simulink model "reset_demo"  (R2015a)
settings: Solver=ode45  SolverMode=SingleTasking  StartTime=0.0  StopTime=100  RelTol=1e-3
libraries: simulink x2
settings Model: CovMetricSettings=dwe  CovHtmlReporting=off  covSaveCumulativeToWorkspaceVar=off  CovSaveSingleToWorkspaceVar=off  CovExternalEMLEnable=on  Creator=cbrooks  LastModifiedBy=hbourbou
settings DataIOCC: LimitDataPoints=off  SaveFormat=Dataset
settings DebuggingCC: SFUnexpectedBacktrackingDiag=error  SFNoUnconditionalDefaultTransitionDiag=error
settings HardwareCC: ProdBitPerPointer=64  ProdLargestAtomicFloat=Float  ProdIntDivRoundTo=Zero  ProdEndianess=LittleEndian  ProdHWDeviceType=Specified
settings ModelReferenceCC: PropagateSignalLabelsOutOfModel=on
settings GRTTargetCC: TargetLangStandard=C99 (ISO)  GeneratePreprocessorConditionals=Use local settings

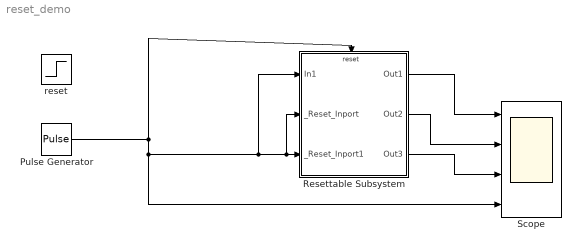
== system reset_demo ==
  Pulse Generator : DiscretePulseGenerator  Period=6  PulseWidth=3
  Resettable Subsystem : Subsystem  TreatAsAtomicUnit=on
  Scope : Scope  NumInputPorts=4
      settings: TimeRange=auto  MaxDataPoints=5000  SaveToWorkspace=off  SaveName=ScopeData  YMin=-0.375~-0.375~-0.375~-0.375  YMax=3.375~3.375~3.375~3.375  SampleTime=-1
  reset : Step  Time=5  SampleTime=.2
  wires:
  Pulse Generator/1 -> Resettable Subsystem/Reset, Scope/4, Resettable Subsystem/1(In1), Resettable Subsystem/2(_Reset_Inport), Resettable Subsystem/3(_Reset_Inport1)
  Resettable Subsystem/1(Out1) -> Scope/1
  Resettable Subsystem/3(Out3) -> Scope/3
  Resettable Subsystem/2(Out2) -> Scope/2

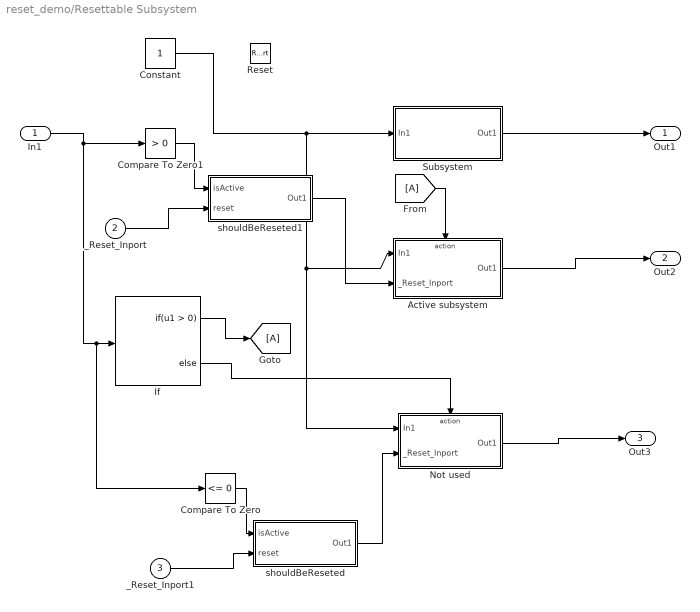
== system reset_demo/Resettable Subsystem ==
  In1 : Inport
  _Reset_Inport : Inport  Port=2
  _Reset_Inport1 : Inport  Port=3
  Reset : ResetPort  DisableCoverage=on  ResetTriggerType=level hold
  Active subsystem : Subsystem  TreatAsAtomicUnit=on
  Compare To Zero : simulink/Logic and Bit Operations/Compare To Zero  relop=<=  OutDataTypeStr=boolean
  Compare To Zero1 : simulink/Logic and Bit Operations/Compare To Zero  relop=>  OutDataTypeStr=boolean
  Constant : Constant  SampleTime=1
  If : If
  Not used : Subsystem  TreatAsAtomicUnit=on
  Subsystem : Subsystem
  shouldBeReseted : Subsystem
  shouldBeReseted1 : Subsystem
  Out1 : Outport
  Out2 : Outport  Port=2
  Out3 : Outport  Port=3
  wires:
  Constant/1 -> Subsystem/1(In1), Not used/1(In1), Active subsystem/1(In1)
  Active subsystem/1(Out1) -> Out2/1
  Subsystem/1(Out1) -> Out1/1
  If/1 -> [A]
  [A] -> Active subsystem/Action
  If/2 -> Not used/Action
  _Reset_Inport/1 -> shouldBeReseted1/2(reset)
  _Reset_Inport1/1 -> shouldBeReseted/2(reset)
  Not used/1(Out1) -> Out3/1
  Compare To Zero/1 -> shouldBeReseted/1(isActive)
  shouldBeReseted/1(Out1) -> Not used/2(_Reset_Inport)
  shouldBeReseted1/1(Out1) -> Active subsystem/2(_Reset_Inport)
  In1/1 -> Compare To Zero1/1, Compare To Zero/1, If/1
  Compare To Zero1/1 -> shouldBeReseted1/1(isActive)

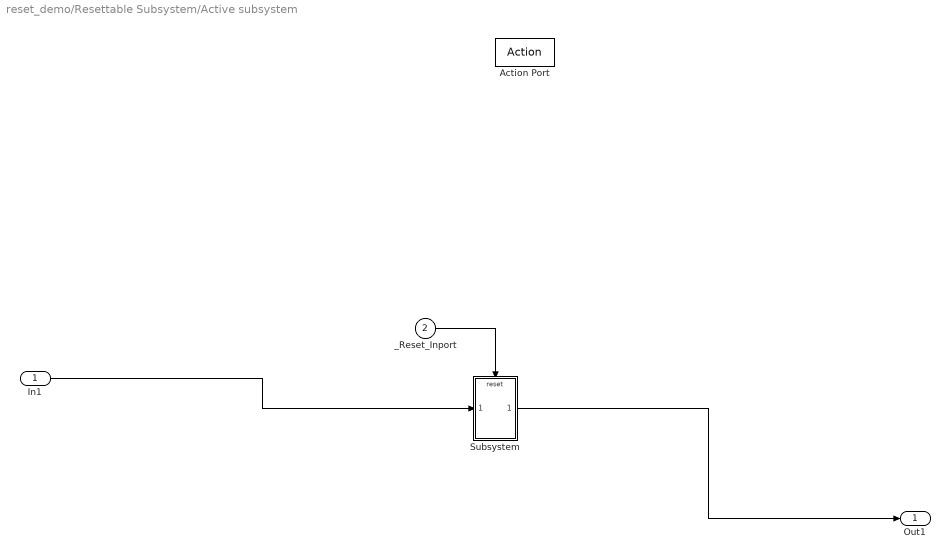
== system reset_demo/Resettable Subsystem/Active subsystem ==
  In1 : Inport
  _Reset_Inport : Inport  Port=2
  Action Port : ActionPort  ActionType=then
  Subsystem : Subsystem
  Out1 : Outport
  wires:
  In1/1 -> Subsystem/1(In1)
  Subsystem/1(Out1) -> Out1/1
  _Reset_Inport/1 -> Subsystem/Reset

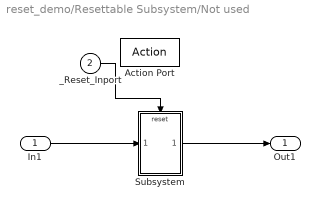
== system reset_demo/Resettable Subsystem/Not used ==
  In1 : Inport
  _Reset_Inport : Inport  Port=2
  Action Port : ActionPort  ActionType=else
  Subsystem : Subsystem
  Out1 : Outport
  wires:
  In1/1 -> Subsystem/1(In1)
  Subsystem/1(Out1) -> Out1/1
  _Reset_Inport/1 -> Subsystem/Reset

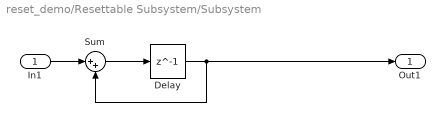
== system reset_demo/Resettable Subsystem/Subsystem ==
  In1 : Inport
  Delay : Delay  DelayLength=1
  Sum : Sum  Inputs=|++
  Out1 : Outport
  wires:
  Delay/1 -> Out1/1, Sum/2
  Sum/1 -> Delay/1
  In1/1 -> Sum/1

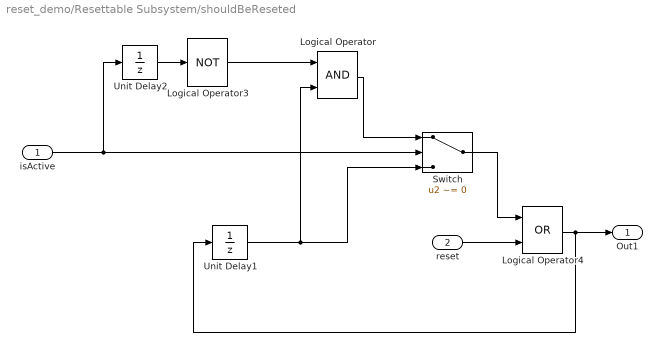
== system reset_demo/Resettable Subsystem/shouldBeReseted ==
  isActive : Inport
  reset : Inport  Port=2
  Logical Operator : Logic  AllPortsSameDT=off  OutDataTypeStr=boolean
  Logical Operator3 : Logic  Operator=NOT  AllPortsSameDT=off  OutDataTypeStr=boolean
  Logical Operator4 : Logic  Operator=OR  AllPortsSameDT=off  OutDataTypeStr=boolean
  Switch : Switch  Criteria=u2 ~= 0
  Unit Delay1 : UnitDelay  SampleTime=-1
  Unit Delay2 : UnitDelay  SampleTime=-1
  Out1 : Outport
  wires:
  isActive/1 -> Switch/2, Unit Delay2/1
  Logical Operator/1 -> Switch/1
  Logical Operator3/1 -> Logical Operator/1
  Unit Delay2/1 -> Logical Operator3/1
  Switch/1 -> Logical Operator4/1
  Logical Operator4/1 -> Unit Delay1/1, Out1/1
  reset/1 -> Logical Operator4/2
  Unit Delay1/1 -> Logical Operator/2, Switch/3

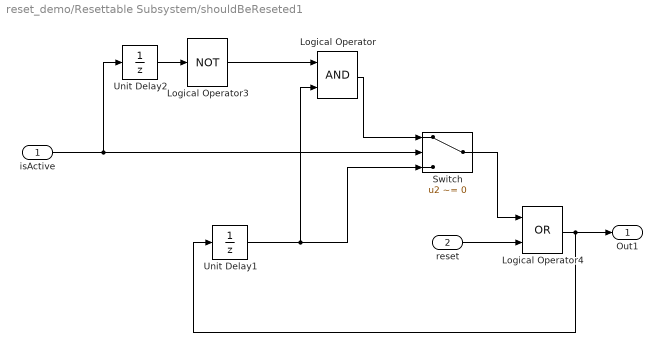
== system reset_demo/Resettable Subsystem/shouldBeReseted1 ==
  isActive : Inport
  reset : Inport  Port=2
  Logical Operator : Logic  AllPortsSameDT=off  OutDataTypeStr=boolean
  Logical Operator3 : Logic  Operator=NOT  AllPortsSameDT=off  OutDataTypeStr=boolean
  Logical Operator4 : Logic  Operator=OR  AllPortsSameDT=off  OutDataTypeStr=boolean
  Switch : Switch  Criteria=u2 ~= 0
  Unit Delay1 : UnitDelay  SampleTime=-1
  Unit Delay2 : UnitDelay  SampleTime=-1
  Out1 : Outport
  wires:
  isActive/1 -> Switch/2, Unit Delay2/1
  Logical Operator/1 -> Switch/1
  Logical Operator3/1 -> Logical Operator/1
  Unit Delay2/1 -> Logical Operator3/1
  Switch/1 -> Logical Operator4/1
  Logical Operator4/1 -> Unit Delay1/1, Out1/1
  reset/1 -> Logical Operator4/2
  Unit Delay1/1 -> Logical Operator/2, Switch/3

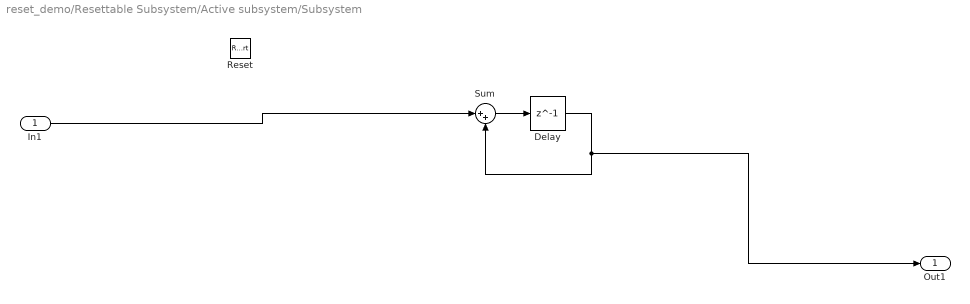
== system reset_demo/Resettable Subsystem/Active subsystem/Subsystem ==
  In1 : Inport
  Reset : ResetPort  DisableCoverage=on  ResetTriggerType=level hold
  Delay : Delay  DelayLength=1
  Sum : Sum  Inputs=|++
  Out1 : Outport
  wires:
  Delay/1 -> Out1/1, Sum/2
  Sum/1 -> Delay/1
  In1/1 -> Sum/1

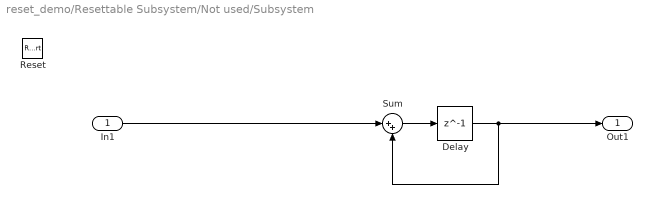
== system reset_demo/Resettable Subsystem/Not used/Subsystem ==
  In1 : Inport
  Reset : ResetPort  DisableCoverage=on  ResetTriggerType=level hold
  Delay : Delay  DelayLength=1
  Sum : Sum  Inputs=|++
  Out1 : Outport
  wires:
  In1/1 -> Sum/1
  Sum/1 -> Delay/1
  Delay/1 -> Sum/2, Out1/1
